simulink model "shj_system_2016a"  (R2016a)
settings: Solver=FixedStepAuto  StartTime=0.0  StopTime=1200  FixedStep=0.02  RelTol=1e-3
values from neighbouring files (symbols this model uses):
  A = 100    [init_shj.m]
  D = 10    [init_nordic.m]    (also in init_shj.m = 50)
  f0 = 50    [init_nordic.m]    (also in init_shj.m)
  H = [3.592 4.602 3.3 3.558 4.925 3.5 3.494 5.403 3.370 7]    [init_nordic.m]    (also in init_shj.m = 3)
  H1 = 2.7    [init_shj.m]
  H2 = A*H    (= 300)    [init_shj.m]
  K11 = bd1*(1-bd1*X22(1,1))    [init_shj.m]
  K12 = bd1*bd2*X22(1,2)    [init_shj.m]
  K13 = bd1*X22(1,3)    [init_shj.m]
  K21 = bd1*bd2*X22(2,1)    [init_shj.m]
  K22 = bd2*(1-bd2*X22(2,2))    [init_shj.m]
  K23 = bd2*X22(2,3)    [init_shj.m]
  Kd = 0.1    [init_shj.m]
  Kd2 = A*Kd    (= 10)    [init_shj.m]
  Kp = 2.5    [PID_parameters.m]    (also in init_nordic.m = 2)
  M1 = 5000    [init_nordic.m]    (also in init_shj.m = 300)
  M2 = 6000    [init_nordic.m]    (also in init_shj.m = 30000)
  R = 0.06    [PID_parameters.m]
  R2 = R    (= 0.06)    [PID_parameters.m]    (also in init_nordic.m = 0.12)
  S_base = 1000    [init_nordic.m]    (also in init_shj.m = 30300)
  Td = 0.6    [PID_parameters.m]    (also in init_nordic.m = 0)
  Tf = 0.2    [PID_parameters.m]    (also in init_nordic.m = 0)
  Ti = 5    [PID_parameters.m]    (also in init_nordic.m)
  Tw = 1.5/2    (= 0.75)    [init_nordic.m]    (also in init_shj.m = 0.6)
  Ty = 0    [init_nordic.m]    (also in init_shj.m = 0.2)
  W0 = 0.01    [init_shj.m]
  Ysp = 0    [init_nordic.m]    (also in init_shj.m)
undefined symbols (not defined in the file or in its folder): ident
settings Model: Creator=sigurdj  LastModifiedBy=sigurd
settings DataIOCC: LimitDataPoints=on  SaveFormat=Array
settings DebuggingCC: SolverPrmCheckMsg=warning
settings HardwareCC: ProdBitPerPointer=32  ProdLargestAtomicFloat=None  ProdIntDivRoundTo=Undefined  ProdEndianess=Unspecified  ProdWordSize=32  ProdHWDeviceType=32-bit Generic
settings ModelReferenceCC: PropagateSignalLabelsOutOfModel=off
settings ConfigComp: CovSFcnEnable=off

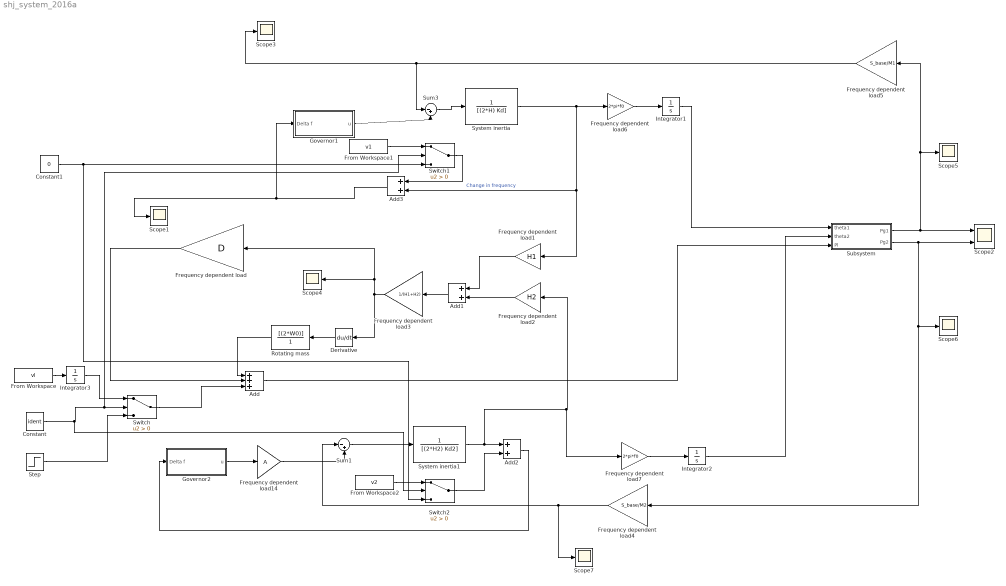
== system shj_system_2016a ==
  Add : Sum  Inputs=+++
  Add1 : Sum
  Add2 : Sum
  Add3 : Sum
  Constant : Constant  Value=ident
  Constant1 : Constant  Value=0
  Derivative : Derivative
  Frequency dependent load : Gain  Gain=D
  Frequency dependent load1 : Gain  Gain=H1
  Frequency dependent load14 : Gain  Gain=A
  Frequency dependent load2 : Gain  Gain=H2
  Frequency dependent load3 : Gain  Gain=1/(H1+H2)
  Frequency dependent load4 : Gain  Gain=S_base/M2
  Frequency dependent load5 : Gain  Gain=S_base/M1
  Frequency dependent load6 : Gain  Gain=2*pi*f0
  Frequency dependent load7 : Gain  Gain=2*pi*f0
  From Workspace : FromWorkspace  VariableName=vl  SampleTime=0
  From Workspace1 : FromWorkspace  VariableName=v1  SampleTime=0
  From Workspace2 : FromWorkspace  VariableName=v2  SampleTime=0
  Governor1 : Subsystem
  Governor2 : Subsystem
  Integrator1 : Integrator
  Integrator2 : Integrator
  Integrator3 : Integrator
  Rotating mass : TransferFcn  Numerator=[(2*W0)]  Denominator=[1]
  Scope{1,3..7} (6 alike) : Scope
  Scope2 : Scope  NumInputPorts=2
  Step : Step  SampleTime=0
  Subsystem : Subsystem
  Sum1 : Sum  Inputs=|-+
  Sum3 : Sum  Inputs=|-+
  Switch : Switch  Criteria=u2 > Threshold
  Switch1 : Switch  Criteria=u2 > Threshold
  Switch2 : Switch  Criteria=u2 > Threshold
  System inertia : TransferFcn  Denominator=[(2*H) Kd]
  System inertia1 : TransferFcn  Denominator=[(2*H2) Kd2]
  wires:
  Sum3/1 -> System inertia/1
  Governor1/1(u) -> Sum3/2
  Derivative/1 -> Rotating mass/1
  Frequency dependent load2/1 -> Add1/2
  Frequency dependent load1/1 -> Add1/1
  Add1/1 -> Frequency dependent load3/1
  Frequency dependent load3/1 -> Scope4/1, Frequency dependent load/1, Derivative/1
  Integrator2/1 -> Subsystem/2(theta2)
  Add/1 -> Subsystem/3(Pl)
  Governor2/1(u) -> Frequency dependent load14/1
  Sum1/1 -> System inertia1/1
  Subsystem/2(Pg2) -> Scope6/1, Frequency dependent load4/1, Scope2/2
  Subsystem/1(Pg1) -> Scope2/1, Scope5/1, Frequency dependent load5/1
  Frequency dependent load4/1 -> Scope7/1, Sum1/1
  Frequency dependent load6/1 -> Integrator1/1
  Frequency dependent load7/1 -> Integrator2/1
  Add3/1 -> Governor1/1(Delta f), Scope1/1
  System inertia1/1 -> Add2/1, Frequency dependent load7/1, Frequency dependent load2/1
  Add2/1 -> Governor2/1(Delta f)
  Integrator1/1 -> Subsystem/1(theta1)
  System inertia/1 -> Frequency dependent load1/1, Add3/2, Frequency dependent load6/1  "Change in frequency"
  Rotating mass/1 -> Add/1
  Frequency dependent load/1 -> Add/2
  Frequency dependent load5/1 -> Sum3/1, Scope3/1
  Frequency dependent load14/1 -> Sum1/2
  From Workspace2/1 -> Switch2/1
  From Workspace/1 -> Integrator3/1
  Integrator3/1 -> Switch/1
  Switch/1 -> Add/3
  Step/1 -> Switch/3
  From Workspace1/1 -> Switch1/1
  Switch1/1 -> Add3/1
  Constant/1 -> Switch2/2, Switch1/2, Switch/2
  Constant1/1 -> Switch2/3, Switch1/3
  Switch2/1 -> Add2/2

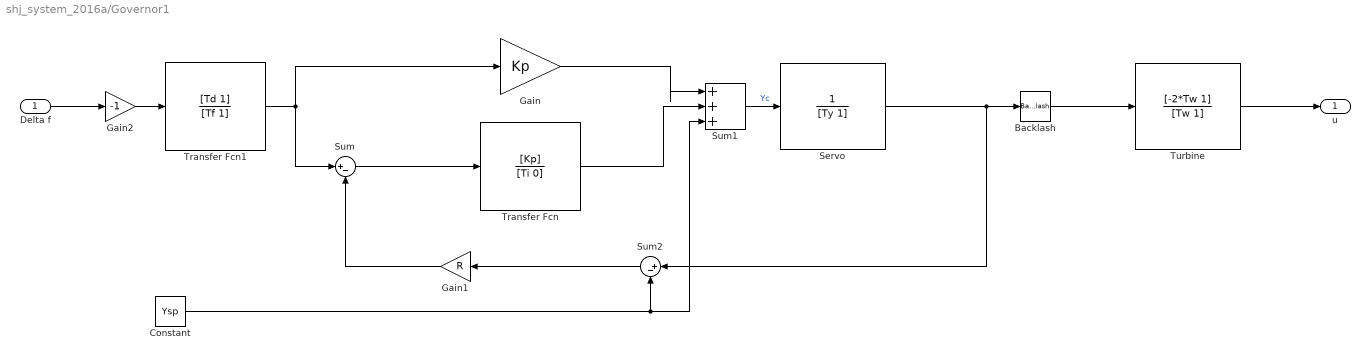
== system shj_system_2016a/Governor1 ==
  Delta f : Inport
  Backlash : Backlash  BacklashWidth=backlash
  Constant : Constant  Value=Ysp
  Gain : Gain  Gain=Kp
  Gain1 : Gain  Gain=R
  Gain2 : Gain  Gain=-1
  Servo : TransferFcn  Denominator=[Ty 1]
  Sum : Sum  Inputs=|+-
  Sum1 : Sum  Inputs=|+++
  Sum2 : Sum  Inputs=|+-
  Transfer Fcn : TransferFcn  Numerator=[Kp]  Denominator=[Ti 0]
  Transfer Fcn1 : TransferFcn  Numerator=[Td 1]  Denominator=[Tf 1]
  Turbine : TransferFcn  Numerator=[-2*Tw 1]  Denominator=[Tw 1]
  u : Outport
  wires:
  Sum/1 -> Transfer Fcn/1
  Delta f/1 -> Gain2/1
  Gain/1 -> Sum1/1
  Transfer Fcn/1 -> Sum1/2
  Gain1/1 -> Sum/2
  Sum1/1 -> Servo/1  "Yc"
  Sum2/1 -> Gain1/1
  Constant/1 -> Sum1/3, Sum2/2
  Backlash/1 -> Turbine/1
  Turbine/1 -> u/1
  Gain2/1 -> Transfer Fcn1/1
  Transfer Fcn1/1 -> Gain/1, Sum/1
  Servo/1 -> Sum2/1, Backlash/1

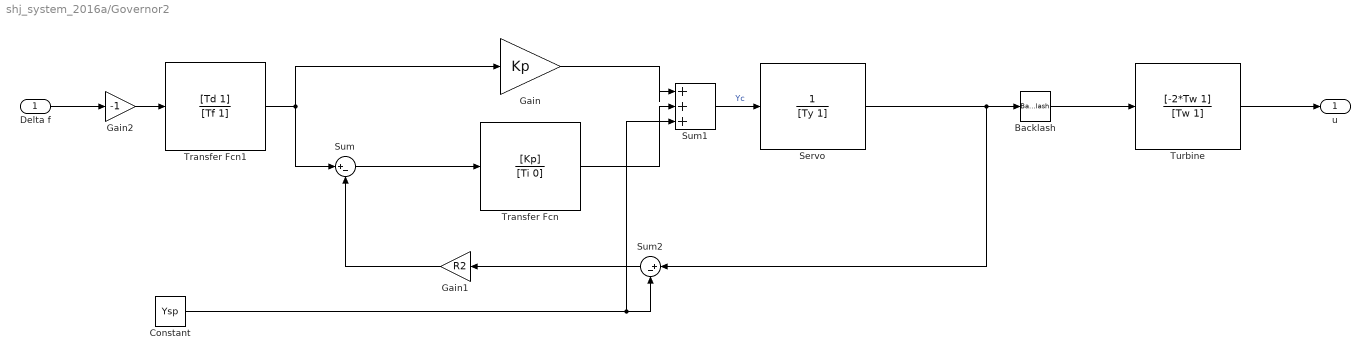
== system shj_system_2016a/Governor2 ==
  Delta f : Inport
  Backlash : Backlash  BacklashWidth=backlash
  Constant : Constant  Value=Ysp
  Gain : Gain  Gain=Kp
  Gain1 : Gain  Gain=R2
  Gain2 : Gain  Gain=-1
  Servo : TransferFcn  Denominator=[Ty 1]
  Sum : Sum  Inputs=|+-
  Sum1 : Sum  Inputs=|+++
  Sum2 : Sum  Inputs=|+-
  Transfer Fcn : TransferFcn  Numerator=[Kp]  Denominator=[Ti 0]
  Transfer Fcn1 : TransferFcn  Numerator=[Td 1]  Denominator=[Tf 1]
  Turbine : TransferFcn  Numerator=[-2*Tw 1]  Denominator=[Tw 1]
  u : Outport
  wires:
  Sum/1 -> Transfer Fcn/1
  Delta f/1 -> Gain2/1
  Gain/1 -> Sum1/1
  Transfer Fcn/1 -> Sum1/2
  Gain1/1 -> Sum/2
  Sum1/1 -> Servo/1  "Yc"
  Sum2/1 -> Gain1/1
  Constant/1 -> Sum2/2, Sum1/3
  Backlash/1 -> Turbine/1
  Turbine/1 -> u/1
  Gain2/1 -> Transfer Fcn1/1
  Transfer Fcn1/1 -> Gain/1, Sum/1
  Servo/1 -> Sum2/1, Backlash/1

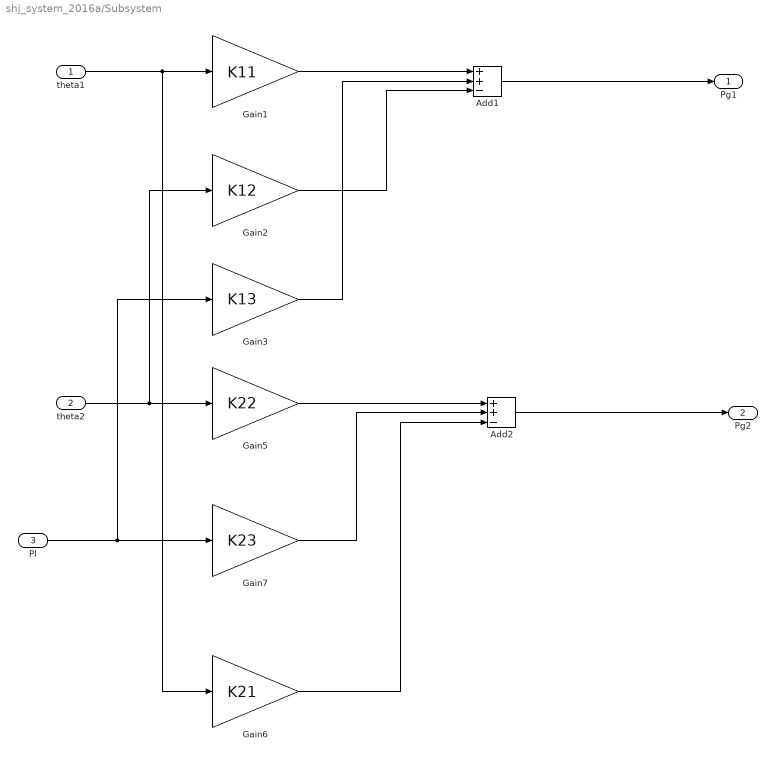
== system shj_system_2016a/Subsystem ==
  theta1 : Inport  PortDimensions=1
  theta2 : Inport  Port=2  PortDimensions=1
  Pl : Inport  Port=3  PortDimensions=1
  Add1 : Sum  Inputs=++-
  Add2 : Sum  Inputs=++-
  Gain1 : Gain  Gain=K11
  Gain2 : Gain  Gain=K12
  Gain3 : Gain  Gain=K13
  Gain5 : Gain  Gain=K22
  Gain6 : Gain  Gain=K21
  Gain7 : Gain  Gain=K23
  Pg1 : Outport
  Pg2 : Outport  Port=2
  wires:
  theta1/1 -> Gain6/1, Gain1/1
  theta2/1 -> Gain5/1, Gain2/1
  Pl/1 -> Gain7/1, Gain3/1
  Gain1/1 -> Add1/1
  Gain2/1 -> Add1/3
  Gain3/1 -> Add1/2
  Add1/1 -> Pg1/1
  Gain6/1 -> Add2/3
  Add2/1 -> Pg2/1
  Gain7/1 -> Add2/2
  Gain5/1 -> Add2/1
